simulink model "PV_Five_Model"  (R2024b)
settings: Solver=VariableStepAuto  StartTime=0.0  StopTime=25  RelTol=1e-3
libraries: simulink x1
settings Model: Creator=86195  LastModifiedBy=86195

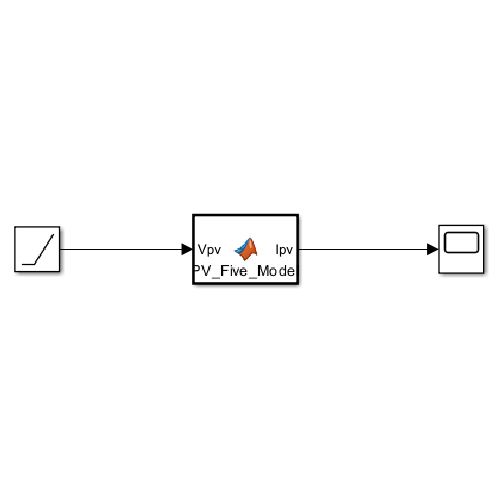
[thumbnail: Simulink's stored preview of the top-level diagram]
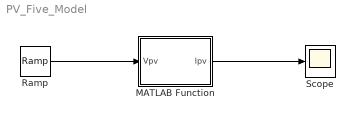
== system PV_Five_Model ==
  MATLAB Function : MATLAB Function  TreatAsAtomicUnit=on
  Ramp : simulink/Sources/Ramp  slope=1  start=0  InitialOutput=0
  Scope : Scope
  wires:
  MATLAB Function/1(Ipv) -> Scope/1
  Ramp/1 -> MATLAB Function/1(Vpv)

== matlab function PV_Five_Model/MATLAB Function ==
  data: Vpv input; Ipv output
function Ipv = PV_Five_Model(Vpv)
%% 光 伏 电 池 五 参 数 模 型 的 搭 建
%% 常 数 量
k = 1.38e-23;
%玻 尔 兹 曼 常 数
q = 1.60e-19;
%单 位 电 荷 量
%% 给 定 参 数
T = 25+273;
%光 伏 电 池 温 度
A = 0.97359;
%二 极 管 的 品 质 因 数
Iph = 3.8;
%光 生 电 流
Is = 2.4515e-10; %二 极 管 反 向 饱 和 电 流
Ns = 36; %光 伏 组 件 串 联 光 伏 单 体 数 量
Rp = 161.0752;
%并 联 电 阻
Rs = 0.38659/Ns;
%串 联 电 阻
%% 公 式
Ipv = zeros(size(Vpv));
%初 始 化
%% 公 式
Vt = k*T/q; %光 伏 电 池 热 电 压
Vpv = Vpv/Ns; %计 算 每 个 串 联 光 伏 单 体 的 电 压
Vd = Vpv+Ipv.*Rs;
Id = Is*(exp(Vd./(A*Vt))-1); %注 意 跟 理 想 模 型 不 同， 此 处 Vd 不 等 于 Vpv
Ip = Vd./Rp;
for i = 1:10 %牛 顿 -拉 夫 逊 法
Ipv = Ipv - (Iph - Ipv - Id - Ip)./(-1 - (Id * Rs./ (A*Vt)) - Rs/Rp);
end
